simulink model "sampleModel7293"  (R2018a)
settings: Solver=VariableStepAuto  StartTime=0.0  StopTime=10.0  RelTol=1e-3
undefined symbols (not defined in the file): DiscIntNeverNeededParam
libraries: simulink x367
(part 1 of 7)
settings Model: Creator=cyfuzz  LastModifiedBy=shafiul
settings CodeAppCC: StateflowObjectComments=on

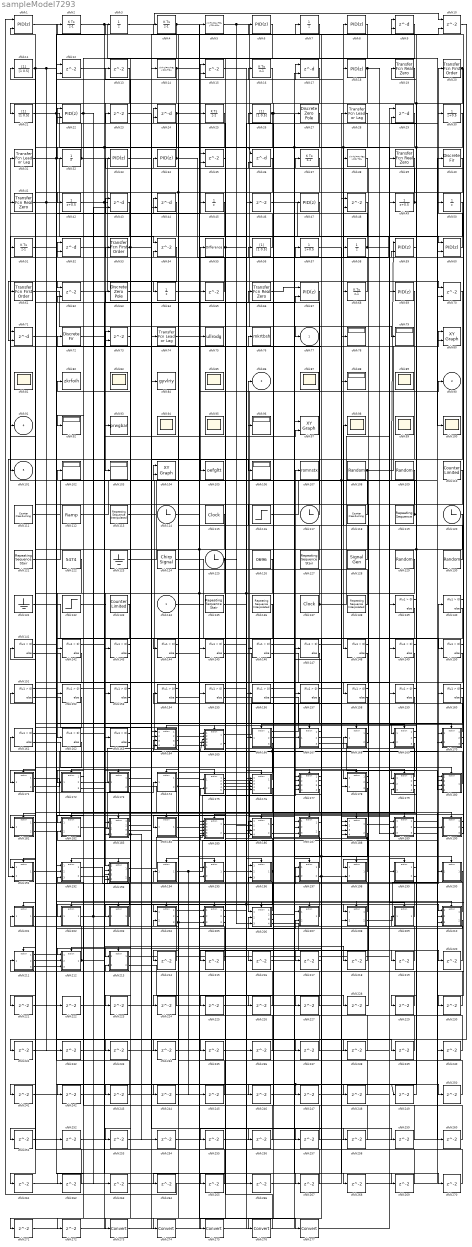
== system sampleModel7293 ==
  cfblk134 : Inport
  cfblk{1,22,59..60,67} (5 alike) : simulink/Continuous/PID Controller (2DOF)  Controller=PID  TimeDomain=Discrete-time  SampleTime=1  IntegratorMethod=Forward Euler  FilterMethod=Forward Euler  Form=Parallel  UseFilter=on  ControllerParametersSource=internal  P=1  I=1  D=0  N=100  b=1  c=1  InitialConditionSource=internal  InitialConditionForIntegrator=0  InitialConditionForFilter=0  ExternalReset=none  LimitOutput=off  UpperSaturationLimit=inf  LowerSaturationLimit=-inf  LinearizeAsGain=off  AntiWindupMode=none  Kb=1  TrackingMode=off  Kt=1  PParamMin=[]  PParamMax=[]  IParamMin=[]  IParamMax=[]  DParamMin=[]  DParamMax=[]  NParamMin=[]  NParamMax=[]  bParamMin=[]  bParamMax=[]  cParamMin=[]  cParamMax=[]  KbParamMin=[]  KbParamMax=[]  KtParamMin=[]  KtParamMax=[]  POutMin=[]  POutMax=[]  IOutMin=[]  IOutMax=[]  DOutMin=[]  DOutMax=[]  NOutMin=[]  NOutMax=[]  bOutMin=[]  bOutMax=[]  cOutMin=[]  cOutMax=[]  KbOutMin=[]  KbOutMax=[]  KtOutMin=[]  KtOutMax=[]  IntegratorOutMin=[]  IntegratorOutMax=[]  FilterOutMin=[]  FilterOutMax=[]  SumOutMin=[]  SumOutMax=[]  Sum1OutMin=[]  Sum1OutMax=[]  Sum2OutMin=[]  Sum2OutMax=[]  Sum3OutMin=[]  Sum3OutMax=[]  SumI1OutMin=[]  SumI1OutMax=[]  SumI2OutMin=[]  SumI2OutMax=[]  SumI3OutMin=[]  SumI3OutMax=[]  SumDOutMin=[]  SumDOutMax=[]  SaturationOutMin=[]  SaturationOutMax=[]  IntegratorContinuousStateAttributes=''  IntegratorStateMustResolveToSignalObject=off  IntegratorRTWStateStorageClass=Auto  FilterContinuousStateAttributes=''  FilterStateMustResolveToSignalObject=off  FilterRTWStateStorageClass=Auto  DifferentiatorICPrevScaledInput=0  DifferentiatorOutMin=[]  DifferentiatorOutMax=[]  FilterDiffOutCoefMin=[]  FilterDiffOutCoefMax=[]  SumDenOutMin=[]  SumDenOutMax=[]  SumNumOutMin=[]  SumNumOutMax=[]  ReciprocalOutMin=[]  ReciprocalOutMax=[]  DivideOutMin=[]  DivideOutMax=[]  TunerSelectOption=Transfer Function Based (PID Tuner App)
  cfblk{10,12,15,35,48,54,62,70,73} (9 alike) : Delay  ShowEnablePort=on  SampleTime=1
      settings: InputPortMap=u0,e6
  cfblk{81,83,85,87,89,94..95,98..100} (10 alike) : Scope
      cfblk81 settings: Floating=on
      cfblk83 settings: Floating=on
      cfblk85 settings: Floating=on
      cfblk87 settings: Floating=on
      cfblk89 settings: Floating=on
      cfblk94 settings: Floating=on
      cfblk95 settings: Floating=on
      cfblk99 settings: Floating=on
  cfblk{78..79,88,92,96,102..103,106} (8 alike) : Display
  cfblk104 : simulink/Sinks/XY Graph  xmin=-1  xmax=1  ymin=-1  ymax=1  st=-1
  cfblk105 : ToWorkspace  VariableName=oefgltt  SaveFormat=Timeseries  SampleTime=-1
  cfblk107 : ToWorkspace  VariableName=romnstx  SaveFormat=Timeseries  SampleTime=-1
  cfblk{108..109,129..130} (4 alike) : RandomNumber  SampleTime=0.1
  cfblk{11,21,26,56} (4 alike) : DiscreteFilter  SampleTime=1
  cfblk110 : simulink/Sources/Counter Limited  uplimit=7  tsamp=-1
  cfblk111 : simulink/Sources/Counter Free-Running  NumBits=16  tsamp=-1
  cfblk112 : simulink/Sources/Ramp  slope=1  start=0  InitialOutput=0
  cfblk113 : simulink/Sources/Repeating Sequence Interpolated  OutValues=[3 1 4 2 1].'  TimeValues=[0 0.1 0.5 0.6 1].'  LookUpMeth=Interpolation-Use End Values  tsamp=0.01  OutMin=[]  OutMax=[]  OutDataTypeStr=double  OutputDataTypeScalingMode=double  OutDataType=fixdt(0,8)  OutScaling=2^-10
  cfblk{114,117,120,125} (4 alike) : Clock
  cfblk115 : DigitalClock
  cfblk116 : Step  After=79  SampleTime=0
  cfblk118 : simulink/Sources/Counter Free-Running  NumBits=16  tsamp=-1
  cfblk119 : simulink/Sources/Repeating Sequence  rep_seq_t=[0 2]  rep_seq_y=[0 2]
  cfblk121 : simulink/Sources/Repeating Sequence Stair  OutValues=[3 1 4 2 1].'  tsamp=-1  OutMin=[]  OutMax=[]  OutDataTypeStr=double  OutputDataTypeScalingMode=double  OutDataType=fixdt(0,8)  ConRadixGroup=Best Precision: Vector-wise  OutScaling=2^-12
  cfblk122 : Constant  Value=5474
  cfblk123 : Ground
  cfblk124 : simulink/Sources/Chirp Signal  f1=0.1  T=100  f2=1
  cfblk126 : Constant  Value=0696
  cfblk127 : simulink/Sources/Repeating Sequence Stair  OutValues=[3 1 4 2 1].'  tsamp=-1  OutMin=[]  OutMax=[]  OutDataTypeStr=double  OutputDataTypeScalingMode=double  OutDataType=fixdt(0,8)  ConRadixGroup=Best Precision: Vector-wise  OutScaling=2^-12
  cfblk128 : SignalGenerator  Units=rad/sec
  cfblk{13,23,46,65,214..272} (63 alike) : Delay  SampleTime=1
  cfblk131 : Ground
  cfblk132 : Step  After=47  SampleTime=0
  cfblk133 : simulink/Sources/Counter Limited  uplimit=7  tsamp=-1
  cfblk135 : simulink/Sources/Repeating Sequence Stair  OutValues=[3 1 4 2 1].'  tsamp=-1  OutMin=[]  OutMax=[]  OutDataTypeStr=double  OutputDataTypeScalingMode=double  OutDataType=fixdt(0,8)  ConRadixGroup=Best Precision: Vector-wise  OutScaling=2^-12
  cfblk136 : simulink/Sources/Repeating Sequence Interpolated  OutValues=[3 1 4 2 1].'  TimeValues=[0 0.1 0.5 0.6 1].'  LookUpMeth=Interpolation-Use End Values  tsamp=0.01  OutMin=[]  OutMax=[]  OutDataTypeStr=double  OutputDataTypeScalingMode=double  OutDataType=fixdt(0,8)  OutScaling=2^-10
  cfblk137 : DigitalClock
  cfblk138 : simulink/Sources/Repeating Sequence Interpolated  OutValues=[3 1 4 2 1].'  TimeValues=[0 0.1 0.5 0.6 1].'  LookUpMeth=Interpolation-Use End Values  tsamp=0.01  OutMin=[]  OutMax=[]  OutDataTypeStr=double  OutputDataTypeScalingMode=double  OutDataType=fixdt(0,8)  OutScaling=2^-10
  cfblk{139..163} (25 alike) : If  SampleTime=1
  cfblk14 : DiscreteStateSpace
  cfblk{2,4,16,25,37,51,68} (7 alike) : DiscreteIntegrator  ICPrevOutput=DiscIntNeverNeededParam  ICPrevScaledInput=DiscIntNeverNeededParam
  cfblk164 : Subsystem  TreatAsAtomicUnit=on
  cfblk165 : Subsystem  TreatAsAtomicUnit=on
  cfblk166 : Subsystem  TreatAsAtomicUnit=on
  cfblk167 : Subsystem  TreatAsAtomicUnit=on
  cfblk168 : Subsystem  TreatAsAtomicUnit=on
  cfblk169 : Subsystem  TreatAsAtomicUnit=on
  cfblk{9,17,24,29,36,43..44,52,71} (9 alike) : Delay  DelayLengthSource=Input port  SampleTime=1
      settings: InputPortMap=u0,p1
  cfblk170 : Subsystem  TreatAsAtomicUnit=on
  cfblk171 : Subsystem  TreatAsAtomicUnit=on
  cfblk172 : Subsystem  TreatAsAtomicUnit=on
  cfblk173 : Subsystem  TreatAsAtomicUnit=on
  cfblk174 : Subsystem  TreatAsAtomicUnit=on
  cfblk175 : Subsystem  TreatAsAtomicUnit=on
  cfblk176 : Subsystem  TreatAsAtomicUnit=on
  cfblk177 : Subsystem  TreatAsAtomicUnit=on
  cfblk178 : Subsystem  TreatAsAtomicUnit=on
  cfblk179 : Subsystem  TreatAsAtomicUnit=on
  cfblk{6,8,18,33..34,47,69} (7 alike) : simulink/Continuous/PID Controller  Controller=PID  TimeDomain=Discrete-time  SampleTime=1  IntegratorMethod=Forward Euler  FilterMethod=Forward Euler  Form=Parallel  UseFilter=on  ControllerParametersSource=internal  P=1  I=1  D=0  N=100  InitialConditionSource=internal  InitialConditionForIntegrator=0  InitialConditionForFilter=0  ExternalReset=none  LimitOutput=off  UpperSaturationLimit=inf  LowerSaturationLimit=-inf  LinearizeAsGain=off  AntiWindupMode=none  Kb=1  TrackingMode=off  Kt=1  PParamMin=[]  PParamMax=[]  IParamMin=[]  IParamMax=[]  DParamMin=[]  DParamMax=[]  NParamMin=[]  NParamMax=[]  KbParamMin=[]  KbParamMax=[]  KtParamMin=[]  KtParamMax=[]  POutMin=[]  POutMax=[]  IOutMin=[]  IOutMax=[]  DOutMin=[]  DOutMax=[]  NOutMin=[]  NOutMax=[]  KbOutMin=[]  KbOutMax=[]  KtOutMin=[]  KtOutMax=[]  IntegratorOutMin=[]  IntegratorOutMax=[]  FilterOutMin=[]  FilterOutMax=[]  SumOutMin=[]  SumOutMax=[]  SumI1OutMin=[]  SumI1OutMax=[]  SumI2OutMin=[]  SumI2OutMax=[]  SumI3OutMin=[]  SumI3OutMax=[]  SumDOutMin=[]  SumDOutMax=[]  SaturationOutMin=[]  SaturationOutMax=[]  IntegratorContinuousStateAttributes=''  IntegratorStateMustResolveToSignalObject=off  IntegratorRTWStateStorageClass=Auto  FilterContinuousStateAttributes=''  FilterStateMustResolveToSignalObject=off  FilterRTWStateStorageClass=Auto  DifferentiatorICPrevScaledInput=0  DifferentiatorOutMin=[]  DifferentiatorOutMax=[]  FilterDiffOutCoefMin=[]  FilterDiffOutCoefMax=[]  SumDenOutMin=[]  SumDenOutMax=[]  SumNumOutMin=[]  SumNumOutMax=[]  ReciprocalOutMin=[]  ReciprocalOutMax=[]  DivideOutMin=[]  DivideOutMax=[]  TunerSelectOption=Transfer Function Based (PID Tuner App)
  cfblk180 : Subsystem  TreatAsAtomicUnit=on
  cfblk181 : Subsystem  TreatAsAtomicUnit=on
  cfblk182 : Subsystem  TreatAsAtomicUnit=on
  cfblk183 : Subsystem  TreatAsAtomicUnit=on
  cfblk184 : Subsystem  TreatAsAtomicUnit=on
  cfblk185 : Subsystem  TreatAsAtomicUnit=on
  cfblk186 : Subsystem  TreatAsAtomicUnit=on
  cfblk187 : Subsystem  TreatAsAtomicUnit=on
  cfblk188 : Subsystem  TreatAsAtomicUnit=on
  cfblk189 : Subsystem  TreatAsAtomicUnit=on
  cfblk{19,39,41,66} (4 alike) : simulink/Discrete/Transfer Fcn Real Zero  ZeroZ=0.75  ICPrevInput=0.0  DoSatur=off
      settings: SourceProductName=Simulink  SourceProductBaseCode=SL
  cfblk190 : Subsystem  TreatAsAtomicUnit=on
  cfblk191 : Subsystem  TreatAsAtomicUnit=on
  cfblk192 : Subsystem  TreatAsAtomicUnit=on
  cfblk193 : Subsystem  TreatAsAtomicUnit=on
  cfblk194 : Subsystem  TreatAsAtomicUnit=on
  cfblk195 : Subsystem  TreatAsAtomicUnit=on
  cfblk196 : Subsystem  TreatAsAtomicUnit=on
  cfblk197 : Subsystem  TreatAsAtomicUnit=on
  cfblk198 : Subsystem  TreatAsAtomicUnit=on
  cfblk199 : Subsystem  TreatAsAtomicUnit=on
  cfblk20 : simulink/Discrete/Transfer Fcn First Order  PoleZ=0.95  ICPrevOutput=0.0  DoSatur=off
      settings: SourceProductName=Simulink
  cfblk200 : Subsystem  TreatAsAtomicUnit=on
  cfblk201 : Subsystem  TreatAsAtomicUnit=on
  cfblk202 : Subsystem  TreatAsAtomicUnit=on
  cfblk203 : Subsystem  TreatAsAtomicUnit=on
  cfblk204 : Subsystem  TreatAsAtomicUnit=on
  cfblk205 : Subsystem  TreatAsAtomicUnit=on
  cfblk206 : Subsystem  TreatAsAtomicUnit=on
  cfblk207 : Subsystem  TreatAsAtomicUnit=on
  cfblk208 : Subsystem  TreatAsAtomicUnit=on
  cfblk209 : Subsystem  TreatAsAtomicUnit=on
  cfblk210 : Subsystem  TreatAsAtomicUnit=on
  cfblk211 : Subsystem  TreatAsAtomicUnit=on
  cfblk212 : Subsystem  TreatAsAtomicUnit=on
  cfblk213 : Subsystem  TreatAsAtomicUnit=on
  cfblk27 : DiscreteZeroPole  Poles=[0 0.5]  Gain=1
  cfblk{273..277} (5 alike) : DataTypeConversion
  cfblk28 : simulink/Discrete/Transfer Fcn Lead or Lag  PoleZ=0.95  ZeroZ=0.75  ICPrevOutput=0.0  ICPrevInput=0.0  DoSatur=off
      settings: SourceProductName=Simulink  SourceProductBaseCode=SL
  cfblk{3,7,32,45,50,58,64} (7 alike) : UnitDelay
  cfblk{30,42,49,57} (4 alike) : DiscreteTransferFcn  SampleTime=1
  cfblk31 : simulink/Discrete/Transfer Fcn Lead or Lag  PoleZ=0.95  ZeroZ=0.75  ICPrevOutput=0.0  ICPrevInput=0.0  DoSatur=off
      settings: SourceProductName=Simulink  SourceProductBaseCode=SL
  cfblk38 : DiscreteStateSpace
  cfblk40 : DiscreteFir  SampleTime=1
  cfblk5 : DiscreteStateSpace
  cfblk53 : simulink/Discrete/Transfer Fcn First Order  PoleZ=0.95  ICPrevOutput=0.0  DoSatur=off
      settings: SourceProductName=Simulink
  cfblk55 : simulink/Discrete/Difference  ICPrevInput=0.0  OutMin=[]  OutMax=[]  OutDataTypeStr=Inherit: Inherit via back propagation  OutDataType=fixdt(1, 16)  OutScaling=2^-10  DoSatur=off
  cfblk61 : simulink/Discrete/Transfer Fcn First Order  PoleZ=0.95  ICPrevOutput=0.0  DoSatur=off
      settings: SourceProductName=Simulink
  cfblk63 : DiscreteZeroPole  Poles=[0 0.5]  Gain=1
  cfblk72 : DiscreteFir  SampleTime=1
  cfblk74 : simulink/Discrete/Transfer Fcn Lead or Lag  PoleZ=0.95  ZeroZ=0.75  ICPrevOutput=0.0  ICPrevInput=0.0  DoSatur=off
      settings: SourceProductName=Simulink  SourceProductBaseCode=SL
  cfblk75 : ToWorkspace  VariableName=ullrodg  SaveFormat=Timeseries  SampleTime=-1
  cfblk76 : ToWorkspace  VariableName=mkrtbsh  SaveFormat=Timeseries  SampleTime=-1
  cfblk80 : simulink/Sinks/XY Graph  xmin=-1  xmax=1  ymin=-1  ymax=1  st=-1
  cfblk82 : ToWorkspace  VariableName=zkrfoih  SaveFormat=Timeseries  SampleTime=-1
  cfblk84 : ToWorkspace  VariableName=gyvlriy  SaveFormat=Timeseries  SampleTime=-1
  cfblk93 : ToWorkspace  VariableName=prwgbar  SaveFormat=Timeseries  SampleTime=-1
  cfblk97 : simulink/Sinks/XY Graph  xmin=-1  xmax=1  ymin=-1  ymax=1  st=-1
  cfblk77 : Outport
  cfblk86 : Outport  Port=2
  cfblk90 : Outport  Port=3
  cfblk91 : Outport  Port=4
  cfblk101 : Outport  Port=5
  wires:
  cfblk129/1 -> cfblk193/1(cfblk1)
  cfblk192/1(cfblk2) -> cfblk140/1
  cfblk123/1 -> cfblk59/1, cfblk78/1
  cfblk119/1 -> cfblk31/1, cfblk59/2
  cfblk112/1 -> cfblk104/1
  cfblk56/1 -> cfblk15/1
  cfblk13/1 -> cfblk103/1
  cfblk14/1 -> cfblk93/1, cfblk150/1
  cfblk34/1 -> cfblk178/1(cfblk1), cfblk22/2
  cfblk210/1(cfblk2) -> cfblk13/1
  cfblk169/1(cfblk2) -> cfblk19/1
  cfblk43/1 -> cfblk101/1
  cfblk164/1(cfblk2) -> cfblk163/1
  cfblk68/1 -> cfblk8/1
  cfblk46/1 -> cfblk60/1
  cfblk48/1 -> cfblk148/1
  cfblk66/1 -> cfblk67/1
  cfblk5/1 -> cfblk77/1, cfblk206/3(cfblk12)
  cfblk172/1(cfblk2) -> cfblk182/1(cfblk1)
  cfblk202/1(cfblk2) -> cfblk43/2, cfblk218/1
  cfblk172/2(cfblk10) -> cfblk5/1
  cfblk62/1 -> cfblk64/1
  cfblk193/1(cfblk2) -> cfblk107/1
  cfblk213/1(cfblk2) -> cfblk49/1
  cfblk111/1 -> cfblk74/1
  cfblk190/1(cfblk2) -> cfblk211/1(cfblk1)
  cfblk132/1 -> cfblk143/1
  cfblk20/1 -> cfblk35/2, cfblk229/1, cfblk230/1
  cfblk174/1(cfblk2) -> cfblk56/1
  cfblk55/1 -> cfblk70/1, cfblk35/1
  cfblk166/1(cfblk2) -> cfblk28/1
  cfblk29/1 -> cfblk68/1, cfblk183/3(cfblk11)
  cfblk138/1 -> cfblk34/1
  cfblk108/1 -> cfblk206/1(cfblk1), cfblk80/2
  cfblk45/1 -> cfblk191/1(cfblk1)
  cfblk209/1(cfblk2) -> cfblk52/1
  cfblk44/1 -> cfblk92/1
  cfblk3/1 -> cfblk10/1
  cfblk31/1 -> cfblk54/1, cfblk146/1
  cfblk181/1(cfblk2) -> cfblk44/1
  cfblk38/1 -> cfblk62/1
  cfblk24/1 -> cfblk32/1, cfblk16/1
  cfblk179/1(cfblk2) -> cfblk41/1
  cfblk136/1 -> cfblk162/1
  cfblk22/1 -> cfblk262/1, cfblk263/1
  cfblk27/1 -> cfblk61/1
  cfblk33/1 -> cfblk208/1(cfblk1)
  cfblk131/1 -> cfblk196/1(cfblk1)
  cfblk178/2(cfblk12) -> cfblk198/1(cfblk1)
  cfblk194/1(cfblk2) -> cfblk190/1(cfblk1), cfblk245/1
  cfblk196/1(cfblk2) -> cfblk202/1(cfblk1), cfblk73/1
  cfblk207/1(cfblk2) -> cfblk63/1
  cfblk8/1 -> cfblk15/2
  cfblk137/1 -> cfblk29/1, cfblk75/1
  cfblk192/2(cfblk11) -> cfblk197/1(cfblk1)
  cfblk203/1(cfblk2) -> cfblk151/1
  cfblk206/1(cfblk2) -> cfblk82/1
  cfblk164/2(cfblk13) -> cfblk90/1
  cfblk11/1 -> cfblk222/1, cfblk250/1, cfblk221/1
  cfblk32/1 -> cfblk100/1, cfblk22/1
  cfblk26/1 -> cfblk216/1, cfblk269/1, cfblk186/3(cfblk6)
  cfblk40/1 -> cfblk42/1
  cfblk201/1(cfblk2) -> cfblk152/1
  cfblk117/1 -> cfblk1/2
  cfblk121/1 -> cfblk27/1
  cfblk109/1 -> cfblk158/1
  cfblk128/1 -> cfblk98/1
  cfblk124/1 -> cfblk187/1(cfblk1)
  cfblk177/1(cfblk2) -> cfblk57/1
  cfblk25/1 -> cfblk213/1(cfblk1)
  cfblk52/1 -> cfblk195/1(cfblk1)
  cfblk127/1 -> cfblk86/1
  cfblk1/1 -> cfblk12/2
  cfblk61/1 -> cfblk79/1
  cfblk175/1(cfblk2) -> cfblk184/1(cfblk1)
  cfblk73/1 -> cfblk173/1(cfblk1)
  cfblk18/1 -> cfblk21/1, cfblk189/3(cfblk13)
  cfblk42/1 -> cfblk84/1, cfblk268/1
  cfblk49/1 -> cfblk24/1, cfblk9/1
  cfblk183/1(cfblk2) -> cfblk11/1
  cfblk166/2(cfblk11) -> cfblk97/1
  cfblk2/1 -> cfblk70/2, cfblk210/1(cfblk1)
  cfblk60/1 -> cfblk20/1
  cfblk175/2(cfblk12) -> cfblk187/2(cfblk8)
  cfblk165/1(cfblk2) -> cfblk88/1
  cfblk185/2(cfblk17) -> cfblk60/2
  cfblk53/1 -> cfblk153/1, cfblk9/2
  cfblk30/1 -> cfblk169/1(cfblk1), cfblk165/5(cfblk13)
  cfblk114/1 -> cfblk205/2(cfblk9)
  cfblk176/1(cfblk2) -> cfblk102/1
  cfblk169/2(cfblk13) -> cfblk53/1
  cfblk4/1 -> cfblk58/1, cfblk172/1(cfblk1)
  cfblk179/2(cfblk13) -> cfblk104/2
  cfblk122/1 -> cfblk142/1
  cfblk65/1 -> cfblk51/1
  cfblk199/2(cfblk11) -> cfblk7/1
  cfblk118/1 -> cfblk55/1
  cfblk198/1(cfblk2) -> cfblk157/1
  cfblk204/1(cfblk2) -> cfblk10/2
  cfblk164/3(cfblk14) -> cfblk71/1
  cfblk130/1 -> cfblk4/1
  cfblk113/1 -> cfblk65/1
  cfblk171/1(cfblk2) -> cfblk199/1(cfblk1)
  cfblk174/2(cfblk9) -> cfblk210/3(cfblk15), cfblk261/1
  cfblk126/1 -> cfblk204/1(cfblk1), cfblk176/4(cfblk10)
  cfblk37/1 -> cfblk241/1, cfblk244/1
  cfblk189/1(cfblk2) -> cfblk180/1(cfblk1)
  cfblk54/1 -> cfblk71/2
  cfblk183/2(cfblk12) -> cfblk67/2
  cfblk206/3(cfblk14) -> cfblk186/1(cfblk1)
  cfblk12/1 -> cfblk205/3(cfblk10), cfblk36/1
  cfblk116/1 -> cfblk50/1
  cfblk164/4(cfblk15) -> cfblk76/1
  cfblk70/1 -> cfblk191/2(cfblk8)
  cfblk180/1(cfblk2) -> cfblk164/3(cfblk11)
  cfblk59/1 -> cfblk29/2
  cfblk182/1(cfblk2) -> cfblk174/1(cfblk1)
  cfblk193/2(cfblk16) -> cfblk212/1(cfblk1)
  cfblk190/2(cfblk7) -> cfblk160/1
  cfblk58/1 -> cfblk169/2(cfblk12), cfblk36/2
  cfblk183/3(cfblk13) -> cfblk45/1
  cfblk28/1 -> cfblk44/2, cfblk177/3(cfblk10)
  cfblk208/1(cfblk2) -> cfblk26/1
  cfblk205/1(cfblk2) -> cfblk30/1
  cfblk169/3(cfblk14) -> cfblk187/3(cfblk9)
  cfblk212/1(cfblk2) -> cfblk96/1, cfblk91/1
  cfblk125/1 -> cfblk171/1(cfblk1), cfblk185/4(cfblk14), cfblk186/2(cfblk5)
  cfblk190/3(cfblk8) -> cfblk37/1
  cfblk204/2(cfblk12) -> cfblk72/1
  cfblk36/1 -> cfblk144/1
  cfblk166/3(cfblk12) -> cfblk203/1(cfblk1), cfblk165/3(cfblk11)
  cfblk205/2(cfblk11) -> cfblk23/1
  cfblk204/3(cfblk13) -> cfblk247/1, cfblk249/1, cfblk62/2
  cfblk135/1 -> cfblk46/1
  cfblk51/1 -> cfblk18/1
  cfblk205/3(cfblk12) -> cfblk182/2(cfblk11)
  cfblk171/2(cfblk9) -> cfblk170/1(cfblk1)
  cfblk134/1 -> cfblk207/1(cfblk1)
  cfblk195/1(cfblk2) -> cfblk210/2(cfblk14), cfblk220/1
  cfblk189/2(cfblk14) -> cfblk170/2(cfblk11)
  cfblk197/1(cfblk2) -> cfblk33/1
  cfblk21/1 -> cfblk139/1, cfblk185/5(cfblk15)
  cfblk183/4(cfblk14) -> cfblk253/1, cfblk254/1
  cfblk211/2(cfblk6) -> cfblk207/2(cfblk7)
  cfblk172/3(cfblk11) -> cfblk66/1
  cfblk133/1 -> cfblk193/3(cfblk14)
  cfblk181/2(cfblk9) -> cfblk80/1
  cfblk211/3(cfblk7) -> cfblk17/1
  cfblk175/5(cfblk15) -> cfblk97/2
  cfblk6/1 -> cfblk105/1
  cfblk23/1 -> cfblk106/1
  cfblk197/2(cfblk15) -> cfblk73/2, cfblk270/1
  cfblk200/1(cfblk2) -> cfblk197/2(cfblk14)
  cfblk170/1(cfblk2) -> cfblk54/2
  cfblk177/2(cfblk12) -> cfblk2/1
  cfblk50/1 -> cfblk193/4(cfblk15)
  cfblk170/2(cfblk12) -> cfblk6/1
  cfblk168/1(cfblk2) -> cfblk48/2
  cfblk41/1 -> cfblk3/1, cfblk232/1
  cfblk168/2(cfblk8) -> cfblk38/1
  cfblk210/2(cfblk16) -> cfblk206/2(cfblk11)
  cfblk188/1(cfblk2) -> cfblk39/1
  cfblk188/2(cfblk12) -> cfblk224/1, cfblk227/1, cfblk186/4(cfblk7)
  cfblk57/1 -> cfblk178/2(cfblk11)
  cfblk177/3(cfblk13) -> cfblk212/2(cfblk8)
  cfblk165/2(cfblk14) -> cfblk43/1
  cfblk115/1 -> cfblk185/2(cfblk12), cfblk183/2(cfblk10)
  cfblk208/2(cfblk13) -> cfblk180/3(cfblk15)
  cfblk170/3(cfblk13) -> cfblk52/2
  cfblk186/2(cfblk8) -> cfblk17/2
  cfblk167/1(cfblk2) -> cfblk212/3(cfblk9)
  cfblk167/2(cfblk15) -> cfblk189/2(cfblk12)
  cfblk167/3(cfblk16) -> cfblk180/4(cfblk16)
  cfblk120/1 -> cfblk181/1(cfblk1), cfblk179/1(cfblk1)
  cfblk189/3(cfblk15) -> cfblk40/1
  cfblk139/1 -> cfblk164/Action
  cfblk139/2 -> cfblk165/Action
  cfblk140/1 -> cfblk166/Action
  cfblk140/2 -> cfblk167/Action
  cfblk141/1 -> cfblk168/Action
  cfblk141/2 -> cfblk169/Action
  cfblk142/1 -> cfblk170/Action
  cfblk142/2 -> cfblk171/Action
  cfblk143/1 -> cfblk172/Action
  cfblk143/2 -> cfblk173/Action
  cfblk144/1 -> cfblk174/Action
  cfblk144/2 -> cfblk175/Action
  cfblk145/1 -> cfblk176/Action
  cfblk145/2 -> cfblk177/Action
  cfblk146/1 -> cfblk178/Action
  cfblk146/2 -> cfblk179/Action
  cfblk147/1 -> cfblk180/Action
  cfblk147/2 -> cfblk181/Action
  cfblk148/1 -> cfblk182/Action
  cfblk148/2 -> cfblk183/Action
  cfblk149/1 -> cfblk184/Action
  cfblk149/2 -> cfblk185/Action
  cfblk150/1 -> cfblk186/Action
  cfblk150/2 -> cfblk187/Action
  cfblk151/1 -> cfblk188/Action
  cfblk151/2 -> cfblk189/Action
  cfblk152/1 -> cfblk190/Action
  cfblk152/2 -> cfblk191/Action
  cfblk153/1 -> cfblk192/Action
  cfblk153/2 -> cfblk193/Action
  cfblk154/1 -> cfblk194/Action
  cfblk154/2 -> cfblk195/Action
  cfblk155/1 -> cfblk196/Action
  cfblk155/2 -> cfblk197/Action
  cfblk156/1 -> cfblk198/Action
  cfblk156/2 -> cfblk199/Action
  cfblk157/1 -> cfblk200/Action
  cfblk157/2 -> cfblk201/Action
  cfblk158/1 -> cfblk202/Action
  cfblk158/2 -> cfblk203/Action
  cfblk159/1 -> cfblk204/Action
  cfblk159/2 -> cfblk205/Action
  cfblk160/1 -> cfblk206/Action
  cfblk160/2 -> cfblk207/Action
  cfblk161/1 -> cfblk208/Action
  cfblk161/2 -> cfblk209/Action
  cfblk162/1 -> cfblk210/Action
  cfblk162/2 -> cfblk211/Action
  cfblk163/1 -> cfblk212/Action
  cfblk163/2 -> cfblk213/Action
  cfblk19/1 -> cfblk214/1
  cfblk214/1 -> cfblk12/1
  cfblk178/1(cfblk2) -> cfblk215/1
  cfblk215/1 -> cfblk205/1(cfblk1)
  cfblk216/1 -> cfblk167/1(cfblk1)
  cfblk15/1 -> cfblk217/1
  cfblk217/1 -> cfblk147/1
  cfblk218/1 -> cfblk175/1(cfblk1)
  cfblk184/1(cfblk2) -> cfblk219/1
  cfblk219/1 -> cfblk161/1
  cfblk220/1 -> cfblk183/1(cfblk1)
  cfblk221/1 -> cfblk192/2(cfblk9)
  cfblk222/1 -> cfblk188/4(cfblk11)
  cfblk39/1 -> cfblk223/1
  cfblk223/1 -> cfblk164/1(cfblk1)
  cfblk224/1 -> cfblk213/2(cfblk12)
  cfblk186/1(cfblk2) -> cfblk225/1
  cfblk225/1 -> cfblk48/1
  cfblk17/1 -> cfblk226/1
  cfblk226/1 -> cfblk165/1(cfblk1)
  cfblk227/1 -> cfblk185/3(cfblk13)
  cfblk185/1(cfblk2) -> cfblk228/1
  cfblk228/1 -> cfblk168/1(cfblk1)
  cfblk229/1 -> cfblk189/1(cfblk1)
  cfblk230/1 -> cfblk179/3(cfblk12)
  cfblk10/1 -> cfblk231/1
  cfblk231/1 -> cfblk188/2(cfblk9)
  cfblk232/1 -> cfblk179/2(cfblk11)
  cfblk179/3(cfblk14) -> cfblk233/1
  cfblk233/1 -> cfblk176/1(cfblk1)
  cfblk176/2(cfblk12) -> cfblk234/1
  cfblk234/1 -> cfblk208/2(cfblk12)
  cfblk179/4(cfblk15) -> cfblk235/1
  cfblk235/1 -> cfblk175/2(cfblk11)
  cfblk236/1 -> cfblk194/1(cfblk1)
  cfblk211/1(cfblk2) -> cfblk237/1
  cfblk237/1 -> cfblk177/1(cfblk1)
  cfblk63/1 -> cfblk238/1
  cfblk238/1 -> cfblk154/1
  cfblk206/2(cfblk13) -> cfblk239/1
  cfblk239/1 -> cfblk185/1(cfblk1)
  cfblk206/4(cfblk15) -> cfblk240/1
  cfblk240/1 -> cfblk177/2(cfblk9)
  cfblk241/1 -> cfblk156/1
  cfblk199/1(cfblk2) -> cfblk242/1
  cfblk242/1 -> cfblk198/2(cfblk13)
  cfblk7/1 -> cfblk243/1
  cfblk243/1 -> cfblk192/1(cfblk1)
  cfblk244/1 -> cfblk195/2(cfblk7)
  cfblk245/1 -> cfblk204/2(cfblk11)
  cfblk72/1 -> cfblk246/1
  cfblk246/1 -> cfblk149/1
  cfblk247/1 -> cfblk188/3(cfblk10)
  cfblk64/1 -> cfblk248/1
  cfblk248/1 -> cfblk176/2(cfblk8)
  cfblk249/1 -> cfblk209/1(cfblk1)
  cfblk250/1 -> cfblk185/6(cfblk16)
  cfblk67/1 -> cfblk251/1
  cfblk251/1 -> cfblk159/1
  cfblk191/1(cfblk2) -> cfblk252/1
  cfblk252/1 -> cfblk164/2(cfblk10)
  cfblk253/1 -> cfblk180/2(cfblk14)
  cfblk254/1 -> cfblk165/4(cfblk12)
  cfblk187/1(cfblk2) -> cfblk255/1
  cfblk255/1 -> cfblk166/1(cfblk1)
  cfblk187/2(cfblk10) -> cfblk256/1
  cfblk256/1 -> cfblk164/4(cfblk12)
  cfblk175/3(cfblk13) -> cfblk257/1
  cfblk257/1 -> cfblk24/2
  cfblk175/4(cfblk14) -> cfblk258/1
  cfblk258/1 -> cfblk192/3(cfblk10)
  cfblk173/1(cfblk2) -> cfblk259/1
  cfblk259/1 -> cfblk196/2(cfblk9)
  cfblk173/2(cfblk12) -> cfblk260/1
  cfblk260/1 -> cfblk196/3(cfblk10)
  cfblk261/1 -> cfblk155/1
  cfblk262/1 -> cfblk141/1
  cfblk263/1 -> cfblk176/5(cfblk11)
  cfblk16/1 -> cfblk264/1
  cfblk264/1 -> cfblk1/1
  cfblk9/1 -> cfblk265/1
  cfblk265/1 -> cfblk201/1(cfblk1)
  cfblk213/2(cfblk13) -> cfblk266/1
  cfblk266/1 -> cfblk188/1(cfblk1)
  cfblk71/1 -> cfblk267/1
  cfblk267/1 -> cfblk165/2(cfblk10)
  cfblk268/1 -> cfblk200/1(cfblk1)
  cfblk269/1 -> cfblk177/4(cfblk11)
  cfblk270/1 -> cfblk176/3(cfblk9)
  cfblk178/3(cfblk13) -> cfblk271/1
  cfblk271/1 -> cfblk193/2(cfblk13)
  cfblk177/4(cfblk14) -> cfblk272/1
  cfblk272/1 -> cfblk145/1
  cfblk110/1 -> cfblk273/1
  cfblk273/1 -> cfblk14/1
  cfblk47/1 -> cfblk274/1
  cfblk274/1 -> cfblk236/1
  cfblk35/1 -> cfblk275/1
  cfblk275/1 -> cfblk47/1
  cfblk69/1 -> cfblk276/1
  cfblk276/1 -> cfblk25/1
  cfblk74/1 -> cfblk277/1
  cfblk277/1 -> cfblk69/1

== system sampleModel7293/cfblk164 ==
  cfblk1 : Inport
  cfblk10 : Inport  Port=2
  cfblk11 : Inport  Port=3
  cfblk12 : Inport  Port=4
  Action Port : ActionPort  ActionType=then
  cfblk3 : DiscreteIntegrator  SampleTime=-1  ICPrevOutput=DiscIntNeverNeededParam  ICPrevScaledInput=DiscIntNeverNeededParam
  cfblk4 : DiscreteZeroPole  Poles=[0 0.5]  Gain=1  SampleTime=-1
  cfblk5 : simulink/Discrete/Transfer Fcn Real Zero  ZeroZ=0.75  ICPrevInput=0.0  DoSatur=off
      settings: SourceProductName=Simulink  SourceProductBaseCode=SL
  cfblk6 : DiscreteZeroPole  Poles=[0 0.5]  Gain=1  SampleTime=-1
  cfblk7 : Delay  ShowEnablePort=on
      settings: InputPortMap=u0,e6
  cfblk8 : simulink/Discrete/Transfer Fcn Lead or Lag  PoleZ=0.95  ZeroZ=0.75  ICPrevOutput=0.0  ICPrevInput=0.0  DoSatur=off
      settings: SourceProductName=Simulink  SourceProductBaseCode=SL
  cfblk9 : simulink/Discrete/Transfer Fcn Lead or Lag  PoleZ=0.95  ZeroZ=0.75  ICPrevOutput=0.0  ICPrevInput=0.0  DoSatur=off
      settings: SourceProductName=Simulink  SourceProductBaseCode=SL
  cfblk2 : Outport
  cfblk13 : Outport  Port=2
  cfblk14 : Outport  Port=3
  cfblk15 : Outport  Port=4
  wires:
  cfblk7/1 -> cfblk15/1
  cfblk8/1 -> cfblk4/1
  cfblk5/1 -> cfblk13/1
  cfblk11/1 -> cfblk7/1
  cfblk1/1 -> cfblk14/1
  cfblk12/1 -> cfblk7/2, cfblk8/1
  cfblk3/1 -> cfblk2/1
  cfblk10/1 -> cfblk3/1
  cfblk9/1 -> cfblk6/1
  cfblk4/1 -> cfblk9/1
  cfblk6/1 -> cfblk5/1

== system sampleModel7293/cfblk165 ==
  cfblk1 : Inport
  cfblk10 : Inport  Port=2
  cfblk11 : Inport  Port=3
  cfblk12 : Inport  Port=4
  cfblk13 : Inport  Port=5
  Action Port : ActionPort  ActionType=else
  cfblk15 : Subsystem  TreatAsAtomicUnit=on
  cfblk16 : Subsystem  TreatAsAtomicUnit=on
  cfblk17 : Delay
  cfblk3 : simulink/Discrete/Transfer Fcn First Order  PoleZ=0.95  ICPrevOutput=0.0  DoSatur=off
      settings: SourceProductName=Simulink
  cfblk4 : DiscreteZeroPole  Poles=[0 0.5]  Gain=1  SampleTime=-1
  cfblk5 : DiscreteZeroPole  Poles=[0 0.5]  Gain=1  SampleTime=-1
  cfblk6 : DiscreteZeroPole  Poles=[0 0.5]  Gain=1  SampleTime=-1
  cfblk7 : DiscreteStateSpace  SampleTime=-1
  cfblk8 : simulink/Continuous/PID Controller  Controller=PID  TimeDomain=Discrete-time  SampleTime=-1  IntegratorMethod=Forward Euler  FilterMethod=Forward Euler  Form=Parallel  UseFilter=on  ControllerParametersSource=internal  P=1  I=1  D=0  N=100  InitialConditionSource=internal  InitialConditionForIntegrator=0  InitialConditionForFilter=0  ExternalReset=none  LimitOutput=off  UpperSaturationLimit=inf  LowerSaturationLimit=-inf  LinearizeAsGain=off  AntiWindupMode=none  Kb=1  TrackingMode=off  Kt=1  PParamMin=[]  PParamMax=[]  IParamMin=[]  IParamMax=[]  DParamMin=[]  DParamMax=[]  NParamMin=[]  NParamMax=[]  KbParamMin=[]  KbParamMax=[]  KtParamMin=[]  KtParamMax=[]  POutMin=[]  POutMax=[]  IOutMin=[]  IOutMax=[]  DOutMin=[]  DOutMax=[]  NOutMin=[]  NOutMax=[]  KbOutMin=[]  KbOutMax=[]  KtOutMin=[]  KtOutMax=[]  IntegratorOutMin=[]  IntegratorOutMax=[]  FilterOutMin=[]  FilterOutMax=[]  SumOutMin=[]  SumOutMax=[]  SumI1OutMin=[]  SumI1OutMax=[]  SumI2OutMin=[]  SumI2OutMax=[]  SumI3OutMin=[]  SumI3OutMax=[]  SumDOutMin=[]  SumDOutMax=[]  SaturationOutMin=[]  SaturationOutMax=[]  IntegratorContinuousStateAttributes=''  IntegratorStateMustResolveToSignalObject=off  IntegratorRTWStateStorageClass=Auto  FilterContinuousStateAttributes=''  FilterStateMustResolveToSignalObject=off  FilterRTWStateStorageClass=Auto  DifferentiatorICPrevScaledInput=0  DifferentiatorOutMin=[]  DifferentiatorOutMax=[]  InitialConditionSetting=State (most efficient)
  cfblk9 : If  SampleTime=1
  cfblk2 : Outport
  cfblk14 : Outport  Port=2
  wires:
  cfblk6/1 -> cfblk5/1
  cfblk3/1 -> cfblk14/1
  cfblk7/1 -> cfblk9/1
  cfblk16/1(cfblk2) -> cfblk2/1
  cfblk13/1 -> cfblk15/1(cfblk1)
  cfblk10/1 -> cfblk8/1
  cfblk15/1(cfblk2) -> cfblk16/1(cfblk1)
  cfblk12/1 -> cfblk6/1
  cfblk5/1 -> cfblk3/1
  cfblk11/1 -> cfblk4/1
  cfblk9/1 -> cfblk15/Action
  cfblk9/2 -> cfblk16/Action
  cfblk16/2(cfblk15) -> cfblk17/1
  cfblk17/1 -> cfblk7/1

== system sampleModel7293/cfblk166 ==
  cfblk1 : Inport
  Action Port : ActionPort  ActionType=then
  cfblk10 : UnitDelay  SampleTime=-1
  cfblk3 : DiscreteTransferFcn
  cfblk4 : DiscreteFir
  cfblk5 : DiscreteFir
  cfblk6 : UnitDelay  SampleTime=-1
  cfblk7 : simulink/Discrete/Difference  ICPrevInput=0.0  OutMin=[]  OutMax=[]  OutDataTypeStr=Inherit: Inherit via back propagation  OutDataType=fixdt(1, 16)  OutScaling=2^-10  DoSatur=off
  cfblk8 : simulink/Discrete/Transfer Fcn Real Zero  ZeroZ=0.75  ICPrevInput=0.0  DoSatur=off
      settings: SourceProductName=Simulink  SourceProductBaseCode=SL
  cfblk9 : DiscreteFilter
  cfblk2 : Outport
  cfblk11 : Outport  Port=2
  cfblk12 : Outport  Port=3
  wires:
  cfblk9/1 -> cfblk6/1
  cfblk10/1 -> cfblk3/1
  cfblk3/1 -> cfblk4/1
  cfblk6/1 -> cfblk8/1
  cfblk1/1 -> cfblk5/1
  cfblk7/1 -> cfblk11/1
  cfblk5/1 -> cfblk9/1, cfblk2/1, cfblk7/1
  cfblk8/1 -> cfblk10/1
  cfblk4/1 -> cfblk12/1

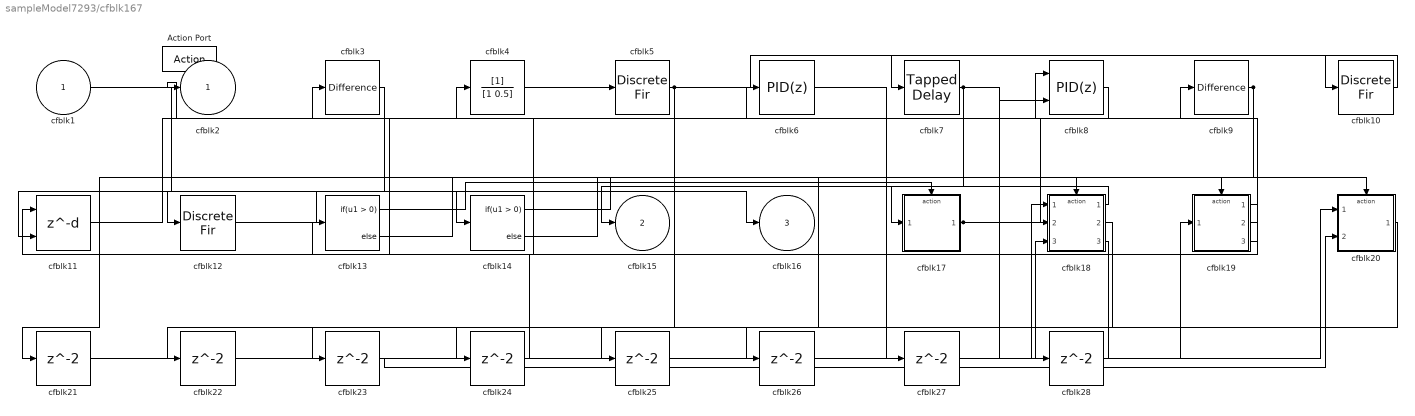
== system sampleModel7293/cfblk167 ==
  cfblk1 : Inport
  Action Port : ActionPort  ActionType=else
  cfblk10 : DiscreteFir
  cfblk11 : Delay  DelayLengthSource=Input port
      settings: InputPortMap=u0,p1
  cfblk12 : DiscreteFir
  cfblk13 : If  SampleTime=1
  cfblk14 : If  SampleTime=1
  cfblk17 : Subsystem  TreatAsAtomicUnit=on
  cfblk18 : Subsystem  TreatAsAtomicUnit=on
  cfblk19 : Subsystem  TreatAsAtomicUnit=on
  cfblk20 : Subsystem  TreatAsAtomicUnit=on
  cfblk{21..28} (8 alike) : Delay
  cfblk3 : simulink/Discrete/Difference  ICPrevInput=0.0  OutMin=[]  OutMax=[]  OutDataTypeStr=Inherit: Inherit via back propagation  OutDataType=fixdt(1, 16)  OutScaling=2^-10  DoSatur=off
  cfblk4 : DiscreteFilter
  cfblk5 : DiscreteFir
  cfblk6 : simulink/Continuous/PID Controller  Controller=PID  TimeDomain=Discrete-time  SampleTime=-1  IntegratorMethod=Forward Euler  FilterMethod=Forward Euler  Form=Parallel  UseFilter=on  ControllerParametersSource=internal  P=1  I=1  D=0  N=100  InitialConditionSource=internal  InitialConditionForIntegrator=0  InitialConditionForFilter=0  ExternalReset=none  LimitOutput=off  UpperSaturationLimit=inf  LowerSaturationLimit=-inf  LinearizeAsGain=off  AntiWindupMode=none  Kb=1  TrackingMode=off  Kt=1  PParamMin=[]  PParamMax=[]  IParamMin=[]  IParamMax=[]  DParamMin=[]  DParamMax=[]  NParamMin=[]  NParamMax=[]  KbParamMin=[]  KbParamMax=[]  KtParamMin=[]  KtParamMax=[]  POutMin=[]  POutMax=[]  IOutMin=[]  IOutMax=[]  DOutMin=[]  DOutMax=[]  NOutMin=[]  NOutMax=[]  KbOutMin=[]  KbOutMax=[]  KtOutMin=[]  KtOutMax=[]  IntegratorOutMin=[]  IntegratorOutMax=[]  FilterOutMin=[]  FilterOutMax=[]  SumOutMin=[]  SumOutMax=[]  SumI1OutMin=[]  SumI1OutMax=[]  SumI2OutMin=[]  SumI2OutMax=[]  SumI3OutMin=[]  SumI3OutMax=[]  SumDOutMin=[]  SumDOutMax=[]  SaturationOutMin=[]  SaturationOutMax=[]  IntegratorContinuousStateAttributes=''  IntegratorStateMustResolveToSignalObject=off  IntegratorRTWStateStorageClass=Auto  FilterContinuousStateAttributes=''  FilterStateMustResolveToSignalObject=off  FilterRTWStateStorageClass=Auto  DifferentiatorICPrevScaledInput=0  DifferentiatorOutMin=[]  DifferentiatorOutMax=[]  InitialConditionSetting=State (most efficient)
  cfblk7 : simulink/Discrete/Tapped Delay  vinit=0.0  samptime=-1  NumDelays=1  DelayOrder=Oldest  includeCurrent=off
  cfblk8 : simulink/Continuous/PID Controller (2DOF)  Controller=PID  TimeDomain=Discrete-time  SampleTime=-1  IntegratorMethod=Forward Euler  FilterMethod=Forward Euler  Form=Parallel  UseFilter=on  ControllerParametersSource=internal  P=1  I=1  D=0  N=100  b=1  c=1  InitialConditionSource=internal  InitialConditionForIntegrator=0  InitialConditionForFilter=0  ExternalReset=none  LimitOutput=off  UpperSaturationLimit=inf  LowerSaturationLimit=-inf  LinearizeAsGain=off  AntiWindupMode=none  Kb=1  TrackingMode=off  Kt=1  PParamMin=[]  PParamMax=[]  IParamMin=[]  IParamMax=[]  DParamMin=[]  DParamMax=[]  NParamMin=[]  NParamMax=[]  bParamMin=[]  bParamMax=[]  cParamMin=[]  cParamMax=[]  KbParamMin=[]  KbParamMax=[]  KtParamMin=[]  KtParamMax=[]  POutMin=[]  POutMax=[]  IOutMin=[]  IOutMax=[]  DOutMin=[]  DOutMax=[]  NOutMin=[]  NOutMax=[]  bOutMin=[]  bOutMax=[]  cOutMin=[]  cOutMax=[]  KbOutMin=[]  KbOutMax=[]  KtOutMin=[]  KtOutMax=[]  IntegratorOutMin=[]  IntegratorOutMax=[]  FilterOutMin=[]  FilterOutMax=[]  SumOutMin=[]  SumOutMax=[]  Sum1OutMin=[]  Sum1OutMax=[]  Sum2OutMin=[]  Sum2OutMax=[]  Sum3OutMin=[]  Sum3OutMax=[]  SumI1OutMin=[]  SumI1OutMax=[]  SumI2OutMin=[]  SumI2OutMax=[]  SumI3OutMin=[]  SumI3OutMax=[]  SumDOutMin=[]  SumDOutMax=[]  SaturationOutMin=[]  SaturationOutMax=[]  IntegratorContinuousStateAttributes=''  IntegratorStateMustResolveToSignalObject=off  IntegratorRTWStateStorageClass=Auto  FilterContinuousStateAttributes=''  FilterStateMustResolveToSignalObject=off  FilterRTWStateStorageClass=Auto  DifferentiatorICPrevScaledInput=0  DifferentiatorOutMin=[]  DifferentiatorOutMax=[]  InitialConditionSetting=State (most efficient)
  cfblk9 : simulink/Discrete/Difference  ICPrevInput=0.0  OutMin=[]  OutMax=[]  OutDataTypeStr=Inherit: Inherit via back propagation  OutDataType=fixdt(1, 16)  OutScaling=2^-10  DoSatur=off
  cfblk2 : Outport
  cfblk15 : Outport  Port=2
  cfblk16 : Outport  Port=3
  wires:
  cfblk1/1 -> cfblk16/1
  cfblk8/1 -> cfblk2/1
  cfblk4/1 -> cfblk5/1
  cfblk17/1(cfblk2) -> cfblk9/1, cfblk8/2
  cfblk19/1(cfblk2) -> cfblk11/1
  cfblk3/1 -> cfblk12/1
  cfblk7/1 -> cfblk17/1(cfblk1), cfblk28/1
  cfblk18/1(cfblk2) -> cfblk15/1
  cfblk10/1 -> cfblk7/1
  cfblk12/1 -> cfblk14/1
  cfblk19/2(cfblk8) -> cfblk13/1
  cfblk5/1 -> cfblk10/1, cfblk11/2
  cfblk19/3(cfblk9) -> cfblk6/1
  cfblk11/1 -> cfblk8/1
  cfblk9/1 -> cfblk21/1, cfblk25/1, cfblk26/1
  cfblk13/1 -> cfblk17/Action
  cfblk13/2 -> cfblk18/Action
  cfblk14/1 -> cfblk19/Action
  cfblk14/2 -> cfblk20/Action
  cfblk21/1 -> cfblk18/1(cfblk1)
  cfblk18/2(cfblk12) -> cfblk22/1
  cfblk22/1 -> cfblk19/1(cfblk1)
  cfblk18/3(cfblk13) -> cfblk23/1
  cfblk23/1 -> cfblk20/2(cfblk7)
  cfblk20/1(cfblk2) -> cfblk24/1
  cfblk24/1 -> cfblk3/1
  cfblk25/1 -> cfblk18/2(cfblk10)
  cfblk26/1 -> cfblk18/3(cfblk11)
  cfblk6/1 -> cfblk27/1
  cfblk27/1 -> cfblk20/1(cfblk1)
  cfblk28/1 -> cfblk4/1

== system sampleModel7293/cfblk168 ==
  cfblk1 : Inport
  Action Port : ActionPort  ActionType=then
  cfblk3 : DiscreteStateSpace  SampleTime=-1
  cfblk4 : simulink/Continuous/PID Controller  Controller=PID  TimeDomain=Discrete-time  SampleTime=-1  IntegratorMethod=Forward Euler  FilterMethod=Forward Euler  Form=Parallel  UseFilter=on  ControllerParametersSource=internal  P=1  I=1  D=0  N=100  InitialConditionSource=internal  InitialConditionForIntegrator=0  InitialConditionForFilter=0  ExternalReset=none  LimitOutput=off  UpperSaturationLimit=inf  LowerSaturationLimit=-inf  LinearizeAsGain=off  AntiWindupMode=none  Kb=1  TrackingMode=off  Kt=1  PParamMin=[]  PParamMax=[]  IParamMin=[]  IParamMax=[]  DParamMin=[]  DParamMax=[]  NParamMin=[]  NParamMax=[]  KbParamMin=[]  KbParamMax=[]  KtParamMin=[]  KtParamMax=[]  POutMin=[]  POutMax=[]  IOutMin=[]  IOutMax=[]  DOutMin=[]  DOutMax=[]  NOutMin=[]  NOutMax=[]  KbOutMin=[]  KbOutMax=[]  KtOutMin=[]  KtOutMax=[]  IntegratorOutMin=[]  IntegratorOutMax=[]  FilterOutMin=[]  FilterOutMax=[]  SumOutMin=[]  SumOutMax=[]  SumI1OutMin=[]  SumI1OutMax=[]  SumI2OutMin=[]  SumI2OutMax=[]  SumI3OutMin=[]  SumI3OutMax=[]  SumDOutMin=[]  SumDOutMax=[]  SaturationOutMin=[]  SaturationOutMax=[]  IntegratorContinuousStateAttributes=''  IntegratorStateMustResolveToSignalObject=off  IntegratorRTWStateStorageClass=Auto  FilterContinuousStateAttributes=''  FilterStateMustResolveToSignalObject=off  FilterRTWStateStorageClass=Auto  DifferentiatorICPrevScaledInput=0  DifferentiatorOutMin=[]  DifferentiatorOutMax=[]  InitialConditionSetting=State (most efficient)
  cfblk5 : DiscreteStateSpace  SampleTime=-1
  cfblk6 : DiscreteFir
  cfblk7 : simulink/Continuous/PID Controller (2DOF)  Controller=PID  TimeDomain=Discrete-time  SampleTime=-1  IntegratorMethod=Forward Euler  FilterMethod=Forward Euler  Form=Parallel  UseFilter=on  ControllerParametersSource=internal  P=1  I=1  D=0  N=100  b=1  c=1  InitialConditionSource=internal  InitialConditionForIntegrator=0  InitialConditionForFilter=0  ExternalReset=none  LimitOutput=off  UpperSaturationLimit=inf  LowerSaturationLimit=-inf  LinearizeAsGain=off  AntiWindupMode=none  Kb=1  TrackingMode=off  Kt=1  PParamMin=[]  PParamMax=[]  IParamMin=[]  IParamMax=[]  DParamMin=[]  DParamMax=[]  NParamMin=[]  NParamMax=[]  bParamMin=[]  bParamMax=[]  cParamMin=[]  cParamMax=[]  KbParamMin=[]  KbParamMax=[]  KtParamMin=[]  KtParamMax=[]  POutMin=[]  POutMax=[]  IOutMin=[]  IOutMax=[]  DOutMin=[]  DOutMax=[]  NOutMin=[]  NOutMax=[]  bOutMin=[]  bOutMax=[]  cOutMin=[]  cOutMax=[]  KbOutMin=[]  KbOutMax=[]  KtOutMin=[]  KtOutMax=[]  IntegratorOutMin=[]  IntegratorOutMax=[]  FilterOutMin=[]  FilterOutMax=[]  SumOutMin=[]  SumOutMax=[]  Sum1OutMin=[]  Sum1OutMax=[]  Sum2OutMin=[]  Sum2OutMax=[]  Sum3OutMin=[]  Sum3OutMax=[]  SumI1OutMin=[]  SumI1OutMax=[]  SumI2OutMin=[]  SumI2OutMax=[]  SumI3OutMin=[]  SumI3OutMax=[]  SumDOutMin=[]  SumDOutMax=[]  SaturationOutMin=[]  SaturationOutMax=[]  IntegratorContinuousStateAttributes=''  IntegratorStateMustResolveToSignalObject=off  IntegratorRTWStateStorageClass=Auto  FilterContinuousStateAttributes=''  FilterStateMustResolveToSignalObject=off  FilterRTWStateStorageClass=Auto  DifferentiatorICPrevScaledInput=0  DifferentiatorOutMin=[]  DifferentiatorOutMax=[]  InitialConditionSetting=State (most efficient)
  cfblk9 : Delay
  cfblk2 : Outport
  cfblk8 : Outport  Port=2
  wires:
  cfblk3/1 -> cfblk6/1
  cfblk4/1 -> cfblk8/1
  cfblk6/1 -> cfblk2/1, cfblk7/1, cfblk7/2
  cfblk1/1 -> cfblk5/1
  cfblk5/1 -> cfblk4/1
  cfblk7/1 -> cfblk9/1
  cfblk9/1 -> cfblk3/1

== system sampleModel7293/cfblk169 ==
  cfblk1 : Inport
  cfblk12 : Inport  Port=2
  Action Port : ActionPort  ActionType=else
  cfblk10 : Delay
  cfblk11 : DiscreteFir
  cfblk3 : DiscreteFilter
  cfblk4 : simulink/Continuous/PID Controller  Controller=PID  TimeDomain=Discrete-time  SampleTime=-1  IntegratorMethod=Forward Euler  FilterMethod=Forward Euler  Form=Parallel  UseFilter=on  ControllerParametersSource=internal  P=1  I=1  D=0  N=100  InitialConditionSource=internal  InitialConditionForIntegrator=0  InitialConditionForFilter=0  ExternalReset=none  LimitOutput=off  UpperSaturationLimit=inf  LowerSaturationLimit=-inf  LinearizeAsGain=off  AntiWindupMode=none  Kb=1  TrackingMode=off  Kt=1  PParamMin=[]  PParamMax=[]  IParamMin=[]  IParamMax=[]  DParamMin=[]  DParamMax=[]  NParamMin=[]  NParamMax=[]  KbParamMin=[]  KbParamMax=[]  KtParamMin=[]  KtParamMax=[]  POutMin=[]  POutMax=[]  IOutMin=[]  IOutMax=[]  DOutMin=[]  DOutMax=[]  NOutMin=[]  NOutMax=[]  KbOutMin=[]  KbOutMax=[]  KtOutMin=[]  KtOutMax=[]  IntegratorOutMin=[]  IntegratorOutMax=[]  FilterOutMin=[]  FilterOutMax=[]  SumOutMin=[]  SumOutMax=[]  SumI1OutMin=[]  SumI1OutMax=[]  SumI2OutMin=[]  SumI2OutMax=[]  SumI3OutMin=[]  SumI3OutMax=[]  SumDOutMin=[]  SumDOutMax=[]  SaturationOutMin=[]  SaturationOutMax=[]  IntegratorContinuousStateAttributes=''  IntegratorStateMustResolveToSignalObject=off  IntegratorRTWStateStorageClass=Auto  FilterContinuousStateAttributes=''  FilterStateMustResolveToSignalObject=off  FilterRTWStateStorageClass=Auto  DifferentiatorICPrevScaledInput=0  DifferentiatorOutMin=[]  DifferentiatorOutMax=[]  InitialConditionSetting=State (most efficient)
  cfblk5 : DiscreteFir
  cfblk6 : Delay  DelayLengthSource=Input port
      settings: InputPortMap=u0,p1
  cfblk7 : DiscreteStateSpace  SampleTime=-1
  cfblk8 : Delay  ShowEnablePort=on
      settings: InputPortMap=u0,e6
  cfblk9 : DiscreteIntegrator  SampleTime=-1  ICPrevOutput=DiscIntNeverNeededParam  ICPrevScaledInput=DiscIntNeverNeededParam
  cfblk2 : Outport
  cfblk13 : Outport  Port=2
  cfblk14 : Outport  Port=3
  wires:
  cfblk1/1 -> cfblk10/1
  cfblk3/1 -> cfblk13/1
  cfblk11/1 -> cfblk8/1
  cfblk5/1 -> cfblk2/1
  cfblk7/1 -> cfblk6/1
  cfblk8/1 -> cfblk5/1
  cfblk9/1 -> cfblk7/1, cfblk4/1
  cfblk12/1 -> cfblk11/1, cfblk8/2, cfblk9/1
  cfblk10/1 -> cfblk6/2
  cfblk4/1 -> cfblk3/1
  cfblk6/1 -> cfblk14/1

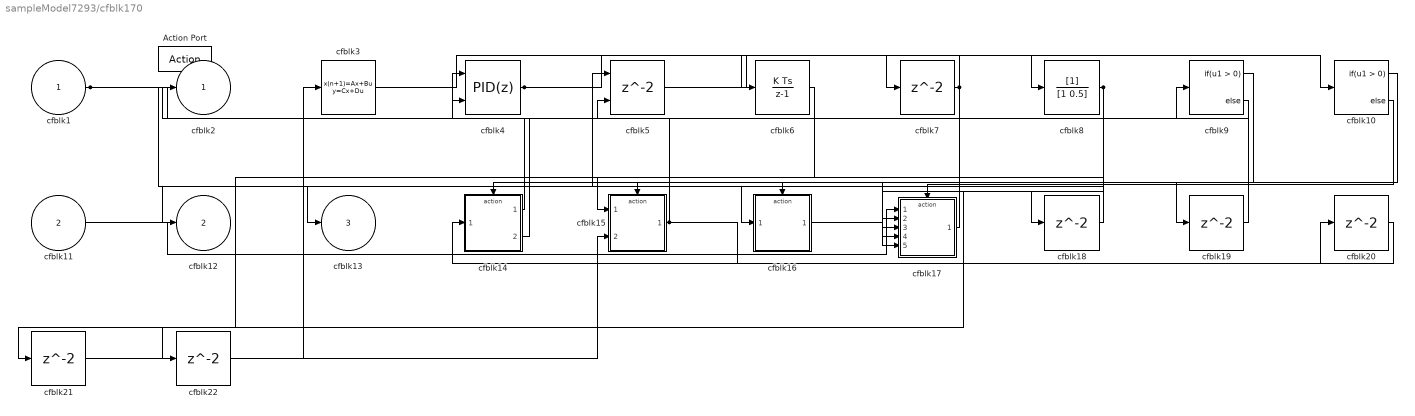
== system sampleModel7293/cfblk170 ==
  cfblk1 : Inport
  cfblk11 : Inport  Port=2
  Action Port : ActionPort  ActionType=then
  cfblk10 : If  SampleTime=1
  cfblk14 : Subsystem  TreatAsAtomicUnit=on
  cfblk15 : Subsystem  TreatAsAtomicUnit=on
  cfblk16 : Subsystem  TreatAsAtomicUnit=on
  cfblk17 : Subsystem  TreatAsAtomicUnit=on
  cfblk{7,18..22} (6 alike) : Delay
  cfblk3 : DiscreteStateSpace  SampleTime=-1
  cfblk4 : simulink/Continuous/PID Controller (2DOF)  Controller=PID  TimeDomain=Discrete-time  SampleTime=-1  IntegratorMethod=Forward Euler  FilterMethod=Forward Euler  Form=Parallel  UseFilter=on  ControllerParametersSource=internal  P=1  I=1  D=0  N=100  b=1  c=1  InitialConditionSource=internal  InitialConditionForIntegrator=0  InitialConditionForFilter=0  ExternalReset=none  LimitOutput=off  UpperSaturationLimit=inf  LowerSaturationLimit=-inf  LinearizeAsGain=off  AntiWindupMode=none  Kb=1  TrackingMode=off  Kt=1  PParamMin=[]  PParamMax=[]  IParamMin=[]  IParamMax=[]  DParamMin=[]  DParamMax=[]  NParamMin=[]  NParamMax=[]  bParamMin=[]  bParamMax=[]  cParamMin=[]  cParamMax=[]  KbParamMin=[]  KbParamMax=[]  KtParamMin=[]  KtParamMax=[]  POutMin=[]  POutMax=[]  IOutMin=[]  IOutMax=[]  DOutMin=[]  DOutMax=[]  NOutMin=[]  NOutMax=[]  bOutMin=[]  bOutMax=[]  cOutMin=[]  cOutMax=[]  KbOutMin=[]  KbOutMax=[]  KtOutMin=[]  KtOutMax=[]  IntegratorOutMin=[]  IntegratorOutMax=[]  FilterOutMin=[]  FilterOutMax=[]  SumOutMin=[]  SumOutMax=[]  Sum1OutMin=[]  Sum1OutMax=[]  Sum2OutMin=[]  Sum2OutMax=[]  Sum3OutMin=[]  Sum3OutMax=[]  SumI1OutMin=[]  SumI1OutMax=[]  SumI2OutMin=[]  SumI2OutMax=[]  SumI3OutMin=[]  SumI3OutMax=[]  SumDOutMin=[]  SumDOutMax=[]  SaturationOutMin=[]  SaturationOutMax=[]  IntegratorContinuousStateAttributes=''  IntegratorStateMustResolveToSignalObject=off  IntegratorRTWStateStorageClass=Auto  FilterContinuousStateAttributes=''  FilterStateMustResolveToSignalObject=off  FilterRTWStateStorageClass=Auto  DifferentiatorICPrevScaledInput=0  DifferentiatorOutMin=[]  DifferentiatorOutMax=[]  InitialConditionSetting=State (most efficient)
  cfblk5 : Delay  ShowEnablePort=on
      settings: InputPortMap=u0,e6
  cfblk6 : DiscreteIntegrator  SampleTime=-1  ICPrevOutput=DiscIntNeverNeededParam  ICPrevScaledInput=DiscIntNeverNeededParam
  cfblk8 : DiscreteFilter
  cfblk9 : If  SampleTime=1
  cfblk2 : Outport
  cfblk12 : Outport  Port=2
  cfblk13 : Outport  Port=3
  wires:
  cfblk5/1 -> cfblk10/1
  cfblk1/1 -> cfblk9/1, cfblk17/5(cfblk13)
  cfblk4/1 -> cfblk8/1, cfblk17/2(cfblk10)
  cfblk17/1(cfblk2) -> cfblk13/1
  cfblk11/1 -> cfblk17/1(cfblk1)
  cfblk3/1 -> cfblk7/1
  cfblk14/1(cfblk2) -> cfblk4/1
  cfblk7/1 -> cfblk16/1(cfblk1), cfblk6/1, cfblk2/1, cfblk17/3(cfblk11)
  cfblk8/1 -> cfblk12/1, cfblk17/4(cfblk12), cfblk18/1, cfblk21/1
  cfblk15/1(cfblk2) -> cfblk5/2, cfblk20/1
  cfblk14/2(cfblk7) -> cfblk4/2
  cfblk9/1 -> cfblk14/Action
  cfblk9/2 -> cfblk15/Action
  cfblk10/1 -> cfblk16/Action
  cfblk10/2 -> cfblk17/Action
  cfblk18/1 -> cfblk15/1(cfblk1)
  cfblk16/1(cfblk2) -> cfblk19/1
  cfblk19/1 -> cfblk5/1
  cfblk20/1 -> cfblk14/1(cfblk1)
  cfblk21/1 -> cfblk15/2(cfblk8)
  cfblk6/1 -> cfblk22/1
  cfblk22/1 -> cfblk3/1

== system sampleModel7293/cfblk171 ==
  cfblk1 : Inport
  Action Port : ActionPort  ActionType=else
  cfblk10 : Subsystem  TreatAsAtomicUnit=on
  cfblk11 : Subsystem  TreatAsAtomicUnit=on
  cfblk{12..15} (4 alike) : Delay
  cfblk3 : DiscreteFilter
  cfblk4 : DiscreteStateSpace  SampleTime=-1
  cfblk5 : DiscreteStateSpace  SampleTime=-1
  cfblk6 : DiscreteStateSpace  SampleTime=-1
  cfblk7 : simulink/Continuous/PID Controller  Controller=PID  TimeDomain=Discrete-time  SampleTime=-1  IntegratorMethod=Forward Euler  FilterMethod=Forward Euler  Form=Parallel  UseFilter=on  ControllerParametersSource=internal  P=1  I=1  D=0  N=100  InitialConditionSource=internal  InitialConditionForIntegrator=0  InitialConditionForFilter=0  ExternalReset=none  LimitOutput=off  UpperSaturationLimit=inf  LowerSaturationLimit=-inf  LinearizeAsGain=off  AntiWindupMode=none  Kb=1  TrackingMode=off  Kt=1  PParamMin=[]  PParamMax=[]  IParamMin=[]  IParamMax=[]  DParamMin=[]  DParamMax=[]  NParamMin=[]  NParamMax=[]  KbParamMin=[]  KbParamMax=[]  KtParamMin=[]  KtParamMax=[]  POutMin=[]  POutMax=[]  IOutMin=[]  IOutMax=[]  DOutMin=[]  DOutMax=[]  NOutMin=[]  NOutMax=[]  KbOutMin=[]  KbOutMax=[]  KtOutMin=[]  KtOutMax=[]  IntegratorOutMin=[]  IntegratorOutMax=[]  FilterOutMin=[]  FilterOutMax=[]  SumOutMin=[]  SumOutMax=[]  SumI1OutMin=[]  SumI1OutMax=[]  SumI2OutMin=[]  SumI2OutMax=[]  SumI3OutMin=[]  SumI3OutMax=[]  SumDOutMin=[]  SumDOutMax=[]  SaturationOutMin=[]  SaturationOutMax=[]  IntegratorContinuousStateAttributes=''  IntegratorStateMustResolveToSignalObject=off  IntegratorRTWStateStorageClass=Auto  FilterContinuousStateAttributes=''  FilterStateMustResolveToSignalObject=off  FilterRTWStateStorageClass=Auto  DifferentiatorICPrevScaledInput=0  DifferentiatorOutMin=[]  DifferentiatorOutMax=[]  InitialConditionSetting=State (most efficient)
  cfblk8 : If  SampleTime=1
  cfblk2 : Outport
  cfblk9 : Outport  Port=2
  wires:
  cfblk7/1 -> cfblk6/1
  cfblk5/1 -> cfblk7/1
  cfblk1/1 -> cfblk11/1(cfblk1)
  cfblk6/1 -> cfblk4/1
  cfblk10/1(cfblk2) -> cfblk3/1
  cfblk11/1(cfblk2) -> cfblk5/1
  cfblk3/1 -> cfblk13/1, cfblk14/1
  cfblk11/2(cfblk8) -> cfblk9/1, cfblk2/1
  cfblk8/1 -> cfblk10/Action
  cfblk8/2 -> cfblk11/Action
  cfblk4/1 -> cfblk12/1
  cfblk12/1 -> cfblk10/1(cfblk1)
  cfblk13/1 -> cfblk11/2(cfblk6)
  cfblk14/1 -> cfblk11/3(cfblk7)
  cfblk10/2(cfblk16) -> cfblk15/1
  cfblk15/1 -> cfblk8/1

== system sampleModel7293/cfblk172 ==
  cfblk1 : Inport
  Action Port : ActionPort  ActionType=then
  cfblk12 : Delay
  cfblk3 : DiscreteFilter
  cfblk4 : simulink/Discrete/Transfer Fcn Lead or Lag  PoleZ=0.95  ZeroZ=0.75  ICPrevOutput=0.0  ICPrevInput=0.0  DoSatur=off
      settings: SourceProductName=Simulink  SourceProductBaseCode=SL
  cfblk5 : Delay  ShowEnablePort=on
      settings: InputPortMap=u0,e6
  cfblk6 : simulink/Discrete/Transfer Fcn First Order  PoleZ=0.95  ICPrevOutput=0.0  DoSatur=off
      settings: SourceProductName=Simulink
  cfblk7 : simulink/Continuous/PID Controller  Controller=PID  TimeDomain=Discrete-time  SampleTime=-1  IntegratorMethod=Forward Euler  FilterMethod=Forward Euler  Form=Parallel  UseFilter=on  ControllerParametersSource=internal  P=1  I=1  D=0  N=100  InitialConditionSource=internal  InitialConditionForIntegrator=0  InitialConditionForFilter=0  ExternalReset=none  LimitOutput=off  UpperSaturationLimit=inf  LowerSaturationLimit=-inf  LinearizeAsGain=off  AntiWindupMode=none  Kb=1  TrackingMode=off  Kt=1  PParamMin=[]  PParamMax=[]  IParamMin=[]  IParamMax=[]  DParamMin=[]  DParamMax=[]  NParamMin=[]  NParamMax=[]  KbParamMin=[]  KbParamMax=[]  KtParamMin=[]  KtParamMax=[]  POutMin=[]  POutMax=[]  IOutMin=[]  IOutMax=[]  DOutMin=[]  DOutMax=[]  NOutMin=[]  NOutMax=[]  KbOutMin=[]  KbOutMax=[]  KtOutMin=[]  KtOutMax=[]  IntegratorOutMin=[]  IntegratorOutMax=[]  FilterOutMin=[]  FilterOutMax=[]  SumOutMin=[]  SumOutMax=[]  SumI1OutMin=[]  SumI1OutMax=[]  SumI2OutMin=[]  SumI2OutMax=[]  SumI3OutMin=[]  SumI3OutMax=[]  SumDOutMin=[]  SumDOutMax=[]  SaturationOutMin=[]  SaturationOutMax=[]  IntegratorContinuousStateAttributes=''  IntegratorStateMustResolveToSignalObject=off  IntegratorRTWStateStorageClass=Auto  FilterContinuousStateAttributes=''  FilterStateMustResolveToSignalObject=off  FilterRTWStateStorageClass=Auto  DifferentiatorICPrevScaledInput=0  DifferentiatorOutMin=[]  DifferentiatorOutMax=[]  InitialConditionSetting=State (most efficient)
  cfblk8 : DiscreteFir
  cfblk9 : simulink/Continuous/PID Controller  Controller=PID  TimeDomain=Discrete-time  SampleTime=-1  IntegratorMethod=Forward Euler  FilterMethod=Forward Euler  Form=Parallel  UseFilter=on  ControllerParametersSource=internal  P=1  I=1  D=0  N=100  InitialConditionSource=internal  InitialConditionForIntegrator=0  InitialConditionForFilter=0  ExternalReset=none  LimitOutput=off  UpperSaturationLimit=inf  LowerSaturationLimit=-inf  LinearizeAsGain=off  AntiWindupMode=none  Kb=1  TrackingMode=off  Kt=1  PParamMin=[]  PParamMax=[]  IParamMin=[]  IParamMax=[]  DParamMin=[]  DParamMax=[]  NParamMin=[]  NParamMax=[]  KbParamMin=[]  KbParamMax=[]  KtParamMin=[]  KtParamMax=[]  POutMin=[]  POutMax=[]  IOutMin=[]  IOutMax=[]  DOutMin=[]  DOutMax=[]  NOutMin=[]  NOutMax=[]  KbOutMin=[]  KbOutMax=[]  KtOutMin=[]  KtOutMax=[]  IntegratorOutMin=[]  IntegratorOutMax=[]  FilterOutMin=[]  FilterOutMax=[]  SumOutMin=[]  SumOutMax=[]  SumI1OutMin=[]  SumI1OutMax=[]  SumI2OutMin=[]  SumI2OutMax=[]  SumI3OutMin=[]  SumI3OutMax=[]  SumDOutMin=[]  SumDOutMax=[]  SaturationOutMin=[]  SaturationOutMax=[]  IntegratorContinuousStateAttributes=''  IntegratorStateMustResolveToSignalObject=off  IntegratorRTWStateStorageClass=Auto  FilterContinuousStateAttributes=''  FilterStateMustResolveToSignalObject=off  FilterRTWStateStorageClass=Auto  DifferentiatorICPrevScaledInput=0  DifferentiatorOutMin=[]  DifferentiatorOutMax=[]  InitialConditionSetting=State (most efficient)
  cfblk2 : Outport
  cfblk10 : Outport  Port=2
  cfblk11 : Outport  Port=3
  wires:
  cfblk3/1 -> cfblk5/1, cfblk2/1
  cfblk5/1 -> cfblk7/1
  cfblk1/1 -> cfblk3/1
  cfblk9/1 -> cfblk8/1, cfblk12/1
  cfblk7/1 -> cfblk11/1
  cfblk4/1 -> cfblk5/2
  cfblk8/1 -> cfblk10/1, cfblk4/1
  cfblk6/1 -> cfblk9/1
  cfblk12/1 -> cfblk6/1
